simulink model "pendulum_animation"  (Simulink 7.2)
settings: Solver=ode45  StartTime=0.0  StopTime=10000  RelTol=1e-3
undefined symbols (not defined in the file or in its folder): drawPendulum
libraries: simulink x2
settings Model: Creator=beard  LastModifiedBy=beard
settings OptimizationCC: InitFltsAndDblsToZero=on

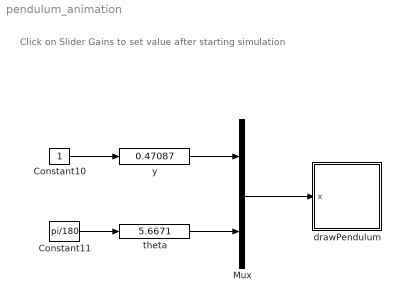
== system pendulum_animation ==
  note: Click on Slider Gains to set value
      | after starting simulation
  Constant10 : Constant  OutDataType=sfix(16)  OutScaling=2^0
  Constant11 : Constant  Value=pi/180  OutDataType=sfix(16)  OutScaling=2^0
  Mux : Mux  Inputs=2
  drawPendulum : Subsystem
      mask init:
      | % drawing parameters
      | L = 1;
      | gap = 0.01;
      | width = 1.0;
      | height = 0.1;
      mask Display: image(imread('tv.jpg'))
  theta : simulink/Math Operations/Slider Gain  SystemSampleTime=-1  low=-180  gain=5.6671  high=180
  y : simulink/Math Operations/Slider Gain  SystemSampleTime=-1  low=-3  gain=0.47087  high=3
  wires:
  y/1 -> Mux/1
  Constant10/1 -> y/1
  theta/1 -> Mux/2
  Constant11/1 -> theta/1
  Mux/1 -> drawPendulum/1(x)

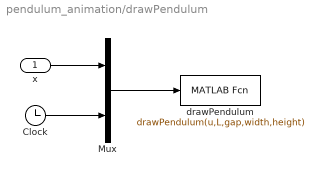
== system pendulum_animation/drawPendulum ==
  x : Inport
  Clock : Clock
      settings: Decimation=10
  Mux : Mux  Inputs=2
  drawPendulum : MATLABFcn  MATLABFcn=drawPendulum(u,L,gap,width,height)  OutputDimensions=0  SampleTime=0.1
  wires:
  Mux/1 -> drawPendulum/1
  x/1 -> Mux/1
  Clock/1 -> Mux/2
